simulink model "W01_Base_MapUnrealPb_cs"  (R2019a)
settings: Solver=FixedStepDiscrete  StartTime=0.0  StopTime=100  FixedStep=1/20  RelTol=1e-3
PreLoadFcn:
  | mbxruntime.callbacks.PreLoadFcn(bdroot);
  | check_NUTS_defined
  | model_closed = 0;
  | assignin('base',['model_closed_' bdroot],false);
PostLoadFcn:
  | mbxruntime.callbacks.PostLoadFcn(bdroot);
InitFcn:
  | mbxruntime.callbacks.InitFcn(bdroot);
StartFcn:
  | mbxruntime.callbacks.StartFcn(bdroot);
StopFcn:
  | mbxruntime.callbacks.StopFcn(bdroot);;
  | 
model workspace: external: MAT-File .\W01_Base_MapUnrealPb_cs_hws.mat (data not in the file)
undefined symbols (not defined in the file or in its folder): DiscIntNeverNeededParam, Header, InitImageOutputDir, mbxruntime, Orientation, Poses, Poses_SL_Info, Position, tabledata, W01_Base_MapUnrealPb_cs_1fa864f6888febdf, W01_Base_MapUnrealPb_cs_363eba12a3b1b1b2, W01_Base_MapUnrealPb_cs_37eda8bac69b475f, W01_Base_MapUnrealPb_cs_40adcda03182ca89, W01_Base_MapUnrealPb_cs_44a3a79c674e7cb2, W01_Base_MapUnrealPb_cs_46a8a6a698ab1958, W01_Base_MapUnrealPb_cs_4b9c3713e3f2fd86, W01_Base_MapUnrealPb_cs_5c6746169321700b, W01_Base_MapUnrealPb_cs_86551b8b23c33892, W01_Base_MapUnrealPb_cs_8a63c705da999788, W01_Base_MapUnrealPb_cs_Audi_A8_Sedan_1_Path_pathUniqueID, W01_Base_MapUnrealPb_cs_c83488546359e010, W01_Base_MapUnrealPb_cs_Child_RegularAni_1_Path_pathUniqueID, W01_Base_MapUnrealPb_cs_Child_RegularAni_2_Path_pathUniqueID, W01_Base_MapUnrealPb_cs_e51f5c648b171aa6, W01_Base_MapUnrealPb_cs_e7dea57c46773520, W01_Base_MapUnrealPb_cs_ea4bc0bfbb614fa1, W01_Base_MapUnrealPb_cs_Female_RegularAni_1_Path_pathUniqueID, W01_Base_MapUnrealPb_cs_Male_RegularAni_1_Path_pathUniqueID, W01_Base_MapUnrealPb_cs_Male_RegularAni_2_Path_pathUniqueID
libraries: adeye_lib x46, simulink_extras x30, simulink x10, robotlib x4, sharedtransform x2, PreScanSimulinkLibrary x2, PreScanUsefulBlocks x1
(part 1 of 9)
CloseFcn:
  | mbxruntime.callbacks.CloseFcn(bdroot);
  | evalin('base',['clear model_closed_' bdroot]);
  | model_closed = 1;
settings Model: Creator=PRESCAN  LastModifiedBy=adeye
settings DataIOCC: LimitDataPoints=on  SaveFormat=Array  SignalLoggingSaveFormat=ModelDataLogs  ReturnWorkspaceOutputs=off
settings OptimizationCC: DefaultParameterBehavior=Inlined  ExpressionDepthLimit=2147483647  InitFltsAndDblsToZero=on  LifeSpan=inf
settings DebuggingCC: SaveWithParameterizedLinksMsg=none  UnderspecifiedInitializationDetection=Classic  MergeDetectMultiDrivingBlocksExec=none  SignalResolutionControl=TryResolveAllWithWarning  MultiTaskDSMMsg=warning  MultiTaskCondExecSysMsg=none  FcnCallInpInsideContextMsg=warning  StateNameClashWarn=warning  SFUnexpectedBacktrackingDiag=warning  SFNoUnconditionalDefaultTransitionDiag=warning  SFExecutionAtInitializationDiag=none  ArithmeticOperatorsInVariantConditions=warning
settings HardwareCC: ProdBitPerPointer=32  ProdBitPerSizeT=32  ProdBitPerPtrDiffT=32  ProdLargestAtomicFloat=None  ProdIntDivRoundTo=Undefined  ProdEndianess=Unspecified  ProdWordSize=32  ProdHWDeviceType=32-bit Generic
settings ModelReferenceCC: UpdateModelReferenceTargets=IfOutOfDate  PropagateSignalLabelsOutOfModel=off
settings SFSimCC: SimUseLocalCustomCode=off  SimParseCustomCode=off
settings SFSimCC: SimCustomHeaderCode=|
  | #include "prescan.h"
  | #include "prescan_platform.h"
  | #include "prescan_aimsunturnindicatorsetter_data.h"
settings RTWCC: RTWUseLocalCustomCode=off
settings CodeAppCC: StateflowObjectComments=on
settings GRTTargetCC: TargetFcnLib=ansi_tfl_tmw.mat  TargetLangStandard=C89/C90 (ANSI)  GeneratePreprocessorConditionals=Disable all  CombineOutputUpdateFcns=off  GRTInterface=on
settings ConfigComp: CovMetricSettings=dw  CovHtmlReporting=on  CovSaveCumulativeToWorkspaceVar=on  CovSaveSingleToWorkspaceVar=on  CovExternalEMLEnable=off  CovSFcnEnable=off

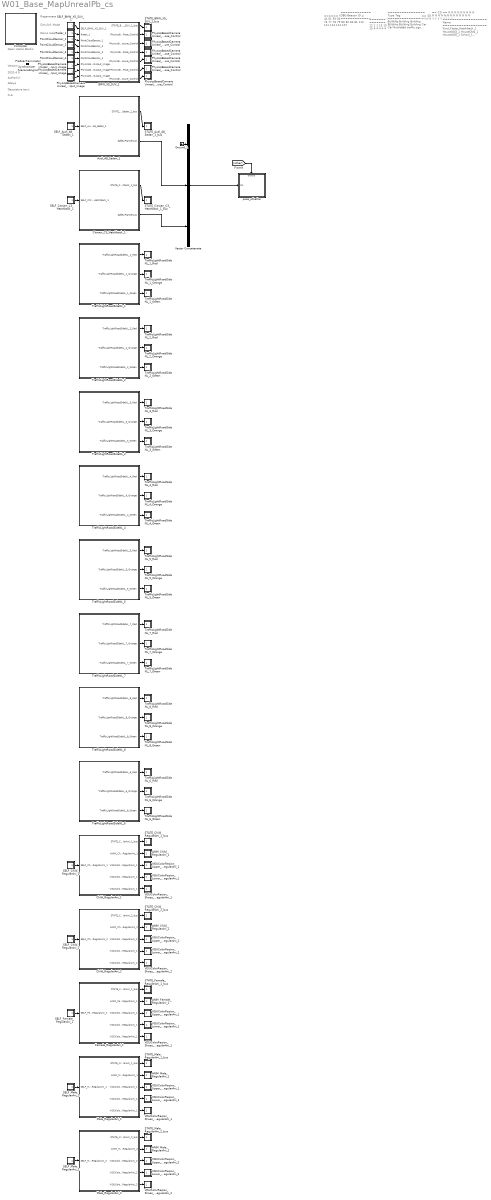
== system W01_Base_MapUnrealPb_cs ==
  note: Regenerate
  note: Simulink Mode
  note: Open Useful Blocks
  note: 2020.4.0
  note: Version:
  note: Author(s):
  note: Adeye
  note: Descriptive text:
  note: N.A.
  note: Demo Help
  note: ======
      | Num ID
      | ======
      | 44
      | 91
      | 93
      | 94
      | 95
      | 96
      | 97
      | 102
      | 108
      | 76
      | 77
      | 78
      | 79
      | 80
      | 82
      | 83
      | 81
      | 112
      | 111
      | 113
      | 114
      | 107
  note: =============
      | OBU-Beacon ID
      | =============
  note: =======
      | Type ID
      | =======
      | 1
      | 12
      | 12
      | 12
      | 12
      | 12
      | 12
      | 1
      | 1
      | 15
      | 15
      | 15
      | 15
      | 15
      | 15
      | 15
      | 15
      | 4
      | 4
      | 4
      | 4
      | 4
  note: ================
      | Type Tag
      | ================
      | Car
      | Building
      | Building
      | Building
      | Building
      | Building
      | Building
      | Car
      | Car
      | Animated traffic sign
      | Animated traffic sign
      | Animated traffic sign
      | Animated traffic sign
      | Animated traffic sign
      | Animated traffic sign
      | Animated traffic sign
      | Animated traffic sign
      | Human
      | Human
      | Human
      | Human
      | Human
  note: ==
      | SD
      | ==
      | Y
      | Y
      | Y
      | Y
      | Y
      | Y
      | Y
      | Y
      | Y
      | Y
      | Y
      | Y
      | Y
      | Y
      | Y
      | Y
      | Y
      | Y
      | Y
      | Y
      | Y
      | Y
  note: ==
      | CD
      | ==
      | N
      | N
      | N
      | N
      | N
      | N
      | N
      | N
      | N
      | N
      | N
      | N
      | N
      | N
      | N
      | N
      | N
      | N
      | N
      | N
      | N
      | N
  note: ===================
      | Name
      | ===================
      | Ford_Fiesta_Hatchback_1
      | HouseOld3_1
      | HouseOld4_1
      | HouseOld5_1
      | School_1
      | OfficeBrownFlat_1
      | OfficeBrownTall2_1
      | Audi_A8_Sedan_1
      | Citroen_C3_Hatchback_1
      | TrafficLightRoadSideNL_1
      | TrafficLightRoadSideNL_2
      | TrafficLightRoadSideNL_3
      | TrafficLightRoadSideNL_4
      | TrafficLightRoadSideNL_5
      | TrafficLightRoadSideNL_7
      | TrafficLightRoadSideNL_8
      | TrafficLightRoadSideNL_6
      | Child_RegularAni_1
      | Child_RegularAni_2
      | Female_RegularAni_1
      | Male_RegularAni_1
      | Male_RegularAni_2
  ANIM_Child_RegularAni_1 : Subsystem  Tag=actuator/AnimationOutport  Priority=0  LoadFcn=load('PreScanAnimActuatorData.mat')  mask(PreScan Sink Block: State Animation){}
      mask help: The Human Animation port allows the human to walk, run or bend
      settings: OpenFcn=open_system([gcb '/Actuator'],'mask')
      mask Help: eval('openHelp(239)')
      mask Display: image(imread('HumanAnimated.jpg'))
  ANIM_Child_RegularAni_2 : Subsystem  Tag=actuator/AnimationOutport  Priority=0  LoadFcn=load('PreScanAnimActuatorData.mat')  mask(PreScan Sink Block: State Animation){}
      mask help: The Human Animation port allows the human to walk, run or bend
      settings: OpenFcn=open_system([gcb '/Actuator'],'mask')
      mask Help: eval('openHelp(239)')
      mask Display: image(imread('HumanAnimated.jpg'))
  ANIM_Female_RegularAni_1 : Subsystem  Tag=actuator/AnimationOutport  Priority=0  LoadFcn=load('PreScanAnimActuatorData.mat')  mask(PreScan Sink Block: State Animation){}
      mask help: The Human Animation port allows the human to walk, run or bend
      settings: OpenFcn=open_system([gcb '/Actuator'],'mask')
      mask Help: eval('openHelp(239)')
      mask Display: image(imread('HumanAnimated.jpg'))
  ANIM_Male_RegularAni_1 : Subsystem  Tag=actuator/AnimationOutport  Priority=0  LoadFcn=load('PreScanAnimActuatorData.mat')  mask(PreScan Sink Block: State Animation){}
      mask help: The Human Animation port allows the human to walk, run or bend
      settings: OpenFcn=open_system([gcb '/Actuator'],'mask')
      mask Help: eval('openHelp(239)')
      mask Display: image(imread('HumanAnimated.jpg'))
  ANIM_Male_RegularAni_2 : Subsystem  Tag=actuator/AnimationOutport  Priority=0  LoadFcn=load('PreScanAnimActuatorData.mat')  mask(PreScan Sink Block: State Animation){}
      mask help: The Human Animation port allows the human to walk, run or bend
      settings: OpenFcn=open_system([gcb '/Actuator'],'mask')
      mask Help: eval('openHelp(239)')
      mask Display: image(imread('HumanAnimated.jpg'))
  Audi_A8_Sedan_1 : Subsystem  Tag=WorldObjectSubSystem  InitFcn=UniqueId = '18645';
      mask init:
      | modelPath = GenericModelHelper.getGenericModelFilePath('ModelDepo','Vehicles\Audi_A8\Audi_A8.pgmb','e33fe1ddcf3e8ae97caccbc8f2fa74ac');imagePath = GenericModelHelper.getCompilationPicture(modelPath, 'Audi_A8_HighPoly.png');
      mask Display: image(imread(imagePath));color('white');text(0, 0, ' ID=102\n')
  BMW_X5_SUV_1 : Subsystem  Tag=WorldObjectSubSystem  InitFcn=UniqueId = '9040';
      mask init:
      | modelPath = GenericModelHelper.getGenericModelFilePath('ModelDepo','Vehicles\BMW_X5\BMW_X5.pgmb','bfeb1c11467705ab888b3011684c848b');imagePath = GenericModelHelper.getCompilationPicture(modelPath, 'BMW_X5_HighPoly.png');
      mask Display: image(imread(imagePath));color('white');text(0, 0, ' ID=55\n')
  Child_RegularAni_1 : Subsystem  Tag=WorldObjectSubSystem  InitFcn=UniqueId = '18395';
      mask init:
      | modelPath = GenericModelHelper.getGenericModelFilePath('ModelDepo','Humans\ChildRegular\Child_Regular.pgmb','0405fb6e1c51d7af34e60031bef9e83f');imagePath = GenericModelHelper.getCompilationPicture(modelPath, 'ChildRegular.png');
      mask Display: image(imread(imagePath));color('white');text(0, 0, ' ID=112\n')
  Child_RegularAni_2 : Subsystem  Tag=WorldObjectSubSystem  InitFcn=UniqueId = '18628';
      mask init: same as W01_Base_MapUnrealPb_cs/Child_RegularAni_1
      mask Display: image(imread(imagePath));color('white');text(0, 0, ' ID=111\n')
  Citroen_C3_Hatchback_1 : Subsystem  Tag=WorldObjectSubSystem  InitFcn=UniqueId = '18857';
      mask init:
      | modelPath = GenericModelHelper.getGenericModelFilePath('ModelDepo','Vehicles\Citroen_C3\Citroen_C3.pgmb','e804ced06d50dbfc6a2202ab3ad01b0c');imagePath = GenericModelHelper.getCompilationPicture(modelPath, 'Citroen_C3_HighPoly.png');
      mask Display: image(imread(imagePath));color('white');text(0, 0, ' ID=108\n')
  Controller : Subsystem  Description=8A3CD2955739A82C886C20AE3E253D78460D53180EE2C1B14CC08DF75A70BE77  Priority=-1  LoadFcn=load PreScanControllerData  mask(PreScan Simulation Controller){prescanversion='2020.4.0', ModelReferencing=off, TimeStep=1/20, ControlMode=0, PreScanExecutionMode=on, ControllerCount=0, ControllerIndex=0, ControllerOptions=''}
      mask prompts: prescanversion "PreScan Version"; ModelReferencing "Use Model Referencing"; TimeStep "Upload Period [s]"; ControlMode "Control Mode"; PreScanExecutionMode "Execution Mode"; ControllerCount "Controller Count"; ControllerIndex "Controller Index"; ControllerOptions "Controller Options"
      mask help:
      | Please do not remove this block from the compilation sheet,
      | as it connects the model to the PreScan environment.
      mask init:
      | model = bdroot(gcb);
      | ExperimentFile = mbxruntime.findExperimentFile(model,true); %relative path
      | 
      | [d1, d2, d3, prescandata] = prescan_Settings();
      | ModelDepo = fullfile(prescandata,'ModelDepo'); 
      | 
      | RTmode = mbxruntime.getRTMode(model);
      | 
      | SimulationMode = get_param(bdroot,'SimulationMode');
      | if strcmp(SimulationMode, 'rapid-accelerator')
      |     SimulationMode = 'external';
      | end
      | TargetName = get_param(bdroot,'SystemTargetFile');
      settings: ModelCloseFcn=assignin('base',['model_closed_' bdroot],true);
      mask Help: eval('openHelp(812)')
      mask Display: image(imread('prescanlogo.ico'))
  Female_RegularAni_1 : Subsystem  Tag=WorldObjectSubSystem  InitFcn=UniqueId = '18631';
      mask init:
      | modelPath = GenericModelHelper.getGenericModelFilePath('ModelDepo','Humans\FemaleRegular\Female_Regular.pgmb','a60942a07dc01011c3a5e5a36c910370');imagePath = GenericModelHelper.getCompilationPicture(modelPath, 'FemaleRegular.png');
      mask Display: image(imread(imagePath));color('white');text(0, 0, ' ID=113\n')
  Ground_1 : Ground
  Male_RegularAni_1 : Subsystem  Tag=WorldObjectSubSystem  InitFcn=UniqueId = '18634';
      mask init:
      | modelPath = GenericModelHelper.getGenericModelFilePath('ModelDepo','Humans\MaleRegular\Male_Regular.pgmb','f91824e3173f6a1007ae98b99b2fb1bd');imagePath = GenericModelHelper.getCompilationPicture(modelPath, 'MaleRegular.png');
      mask Display: image(imread(imagePath));color('white');text(0, 0, ' ID=114\n')
  Male_RegularAni_2 : Subsystem  Tag=WorldObjectSubSystem  InitFcn=UniqueId = '18853';
      mask init: same as W01_Base_MapUnrealPb_cs/Male_RegularAni_1
      mask Display: image(imread(imagePath));color('white');text(0, 0, ' ID=107\n')
  PhysicsBasedCameraUnreal_1_ImageRGBOutput_image : Subsystem  Tag=sensor/plugin/sfun_PBCURGBOutput  Priority=30  mask(PreScan Source Block: Camera Sensor){}
      mask help: Unreal Camera ImageRGBOutput image
      settings: OpenFcn=open_system([gcb '/Sensor'],'mask')
      mask Help: eval('openHelp()')
      mask Display: image(imread('CameraSensor.png'))
  PhysicsBasedCameraUnreal_1_PBCUExposure_Control : Subsystem  Tag=actuator/plugin/sfun_PBCUExposure  Priority=0  mask(Physics Based Camera (Unreal) plugin block){}
      mask help: PBCU Control I/O
      settings: OpenFcn=open_system([gcb '/Actuator'],'mask')
      mask Help: eval('openHelp()')
      mask Display: image(imread('ico_PBCUControl.png'))
  PhysicsBasedCameraUnreal_1_PBCUPose_Control : Subsystem  Tag=actuator/plugin/sfun_PBCUPose  Priority=0  mask(Physics Based Camera (Unreal) plugin block){}
      mask help: PBCU Control I/O
      settings: OpenFcn=open_system([gcb '/Actuator'],'mask')
      mask Help: eval('openHelp()')
      mask Display: image(imread('ico_PBCUControl.png'))
  PhysicsBasedCameraUnreal_2_ImageRGBOutput_image : Subsystem  Tag=sensor/plugin/sfun_PBCURGBOutput  Priority=30  mask(PreScan Source Block: Camera Sensor){}
      mask help: Unreal Camera ImageRGBOutput image
      settings: OpenFcn=open_system([gcb '/Sensor'],'mask')
      mask Help: eval('openHelp()')
      mask Display: image(imread('CameraSensor.png'))
  PhysicsBasedCameraUnreal_2_PBCUExposure_Control : Subsystem  Tag=actuator/plugin/sfun_PBCUExposure  Priority=0  mask(Physics Based Camera (Unreal) plugin block){}
      mask help: PBCU Control I/O
      settings: OpenFcn=open_system([gcb '/Actuator'],'mask')
      mask Help: eval('openHelp()')
      mask Display: image(imread('ico_PBCUControl.png'))
  PhysicsBasedCameraUnreal_2_PBCUPose_Control : Subsystem  Tag=actuator/plugin/sfun_PBCUPose  Priority=0  mask(Physics Based Camera (Unreal) plugin block){}
      mask help: PBCU Control I/O
      settings: OpenFcn=open_system([gcb '/Actuator'],'mask')
      mask Help: eval('openHelp()')
      mask Display: image(imread('ico_PBCUControl.png'))
  PhysicsBasedCameraUnreal_3_ImageRGBOutput_image : Subsystem  Tag=sensor/plugin/sfun_PBCURGBOutput  Priority=30  mask(PreScan Source Block: Camera Sensor){}
      mask help: Unreal Camera ImageRGBOutput image
      settings: OpenFcn=open_system([gcb '/Sensor'],'mask')
      mask Help: eval('openHelp()')
      mask Display: image(imread('CameraSensor.png'))
  PhysicsBasedCameraUnreal_3_PBCUExposure_Control : Subsystem  Tag=actuator/plugin/sfun_PBCUExposure  Priority=0  mask(Physics Based Camera (Unreal) plugin block){}
      mask help: PBCU Control I/O
      settings: OpenFcn=open_system([gcb '/Actuator'],'mask')
      mask Help: eval('openHelp()')
      mask Display: image(imread('ico_PBCUControl.png'))
  PhysicsBasedCameraUnreal_3_PBCUPose_Control : Subsystem  Tag=actuator/plugin/sfun_PBCUPose  Priority=0  mask(Physics Based Camera (Unreal) plugin block){}
      mask help: PBCU Control I/O
      settings: OpenFcn=open_system([gcb '/Actuator'],'mask')
      mask Help: eval('openHelp()')
      mask Display: image(imread('ico_PBCUControl.png'))
  PointCloudSensor_1 : Subsystem  Tag=sensor/PointCloudInport  Priority=30  mask(PreScan Source Block: Point Cloud Sensor){}
      mask help: The Point Cloud Sensor provides XYZ positions relative to the sensor
      settings: OpenFcn=open_system([gcb '/Sensor'],'mask')
      mask Help: eval('openHelp(6400)')
      mask Display: image(imread('PointCloudSensorSL.png'))
  PointCloudSensor_2 : Subsystem  Tag=sensor/PointCloudInport  Priority=30  mask(PreScan Source Block: Point Cloud Sensor){}
      mask help: The Point Cloud Sensor provides XYZ positions relative to the sensor
      settings: OpenFcn=open_system([gcb '/Sensor'],'mask')
      mask Help: eval('openHelp(6400)')
      mask Display: image(imread('PointCloudSensorSL.png'))
  PointCloudSensor_3 : Subsystem  Tag=sensor/PointCloudInport  Priority=30  mask(PreScan Source Block: Point Cloud Sensor){}
      mask help: The Point Cloud Sensor provides XYZ positions relative to the sensor
      settings: OpenFcn=open_system([gcb '/Sensor'],'mask')
      mask Help: eval('openHelp(6400)')
      mask Display: image(imread('PointCloudSensorSL.png'))
  PointCloudSensor_4 : Subsystem  Tag=sensor/PointCloudInport  Priority=30  mask(PreScan Source Block: Point Cloud Sensor){}
      mask help: The Point Cloud Sensor provides XYZ positions relative to the sensor
      settings: OpenFcn=open_system([gcb '/Sensor'],'mask')
      mask Help: eval('openHelp(6400)')
      mask Display: image(imread('PointCloudSensorSL.png'))
  PreScanTerminator : Subsystem  Tag=PreScanTerminator  Priority=999  LoadFcn=load PrescanTerminatorData  mask(PreScan Simulation Terminator){TimeStep=1/20}
      mask prompts: TimeStep "Upload Period [s]"
      mask help:
      | Please do not remove this block from the compilation sheet as it
      | connects the model to the PreScan environment.
      mask Help: eval('openHelp(812)')
      mask Display: image(imread('prescanlogo.ico'))
  Radar_1 : Subsystem  Tag=sensor/Radar  Priority=30  LoadFcn=load('PrescanScannerSensorData.mat');load('PrescanScannerSensorMessage.mat')  mask(PreScan Source Block: Radar Sensor){}
      mask help:
      | The Radar Sensor is a detailed sensor based on a physical radar
      | model that includes Antenna GAIN Maps (AGM) and atmospheric
      | attenuation.
      |
      | For more information, please click Help.
      settings: OpenFcn=open_system([gcb '/Sensor'],'mask')
      mask Help: eval('openHelp(1464)')
      mask Display: image(imread('Radar.png'))
  SELF_Audi_A8_Sedan_1 : Subsystem  Tag=sensor/SelfPort  Priority=30  LoadFcn=load('PreScanSelfSensorData.mat')  mask(PreScan Source Block: SELF){}
      mask help:
      | The SELF port shows (state) information of the actor itself. The outputs are position in the experiment's axis system and the GPS coordinates, and the object's absolute velocity and compass heading.
      |
      | For more information, please click Help.
      settings: OpenFcn=open_system([gcb '/Sensor'],'mask')
      mask Help: eval('openHelp(462)')
      mask Display: image(imread('GPS.png'))
  SELF_BMW_X5_SUV_1 : Subsystem  Tag=sensor/SelfPort  Priority=30  LoadFcn=load('PreScanSelfSensorData.mat')  mask(PreScan Source Block: SELF){}
      mask help:
      | The SELF port shows (state) information of the actor itself. The outputs are position in the experiment's axis system and the GPS coordinates, and the object's absolute velocity and compass heading.
      |
      | For more information, please click Help.
      settings: OpenFcn=open_system([gcb '/Sensor'],'mask')
      mask Help: eval('openHelp(462)')
      mask Display: image(imread('GPS.png'))
  SELF_Child_RegularAni_1 : Subsystem  Tag=sensor/SelfPort  Priority=30  LoadFcn=load('PreScanSelfSensorData.mat')  mask(PreScan Source Block: SELF){}
      mask help:
      | The SELF port shows (state) information of the actor itself. The outputs are position in the experiment's axis system and the GPS coordinates, and the object's absolute velocity and compass heading.
      |
      | For more information, please click Help.
      settings: OpenFcn=open_system([gcb '/Sensor'],'mask')
      mask Help: eval('openHelp(462)')
      mask Display: image(imread('GPS.png'))
  SELF_Child_RegularAni_2 : Subsystem  Tag=sensor/SelfPort  Priority=30  LoadFcn=load('PreScanSelfSensorData.mat')  mask(PreScan Source Block: SELF){}
      mask help:
      | The SELF port shows (state) information of the actor itself. The outputs are position in the experiment's axis system and the GPS coordinates, and the object's absolute velocity and compass heading.
      |
      | For more information, please click Help.
      settings: OpenFcn=open_system([gcb '/Sensor'],'mask')
      mask Help: eval('openHelp(462)')
      mask Display: image(imread('GPS.png'))
  SELF_Citroen_C3_Hatchback_1 : Subsystem  Tag=sensor/SelfPort  Priority=30  LoadFcn=load('PreScanSelfSensorData.mat')  mask(PreScan Source Block: SELF){}
      mask help:
      | The SELF port shows (state) information of the actor itself. The outputs are position in the experiment's axis system and the GPS coordinates, and the object's absolute velocity and compass heading.
      |
      | For more information, please click Help.
      settings: OpenFcn=open_system([gcb '/Sensor'],'mask')
      mask Help: eval('openHelp(462)')
      mask Display: image(imread('GPS.png'))
  SELF_Female_RegularAni_1 : Subsystem  Tag=sensor/SelfPort  Priority=30  LoadFcn=load('PreScanSelfSensorData.mat')  mask(PreScan Source Block: SELF){}
      mask help:
      | The SELF port shows (state) information of the actor itself. The outputs are position in the experiment's axis system and the GPS coordinates, and the object's absolute velocity and compass heading.
      |
      | For more information, please click Help.
      settings: OpenFcn=open_system([gcb '/Sensor'],'mask')
      mask Help: eval('openHelp(462)')
      mask Display: image(imread('GPS.png'))
  SELF_Male_RegularAni_1 : Subsystem  Tag=sensor/SelfPort  Priority=30  LoadFcn=load('PreScanSelfSensorData.mat')  mask(PreScan Source Block: SELF){}
      mask help:
      | The SELF port shows (state) information of the actor itself. The outputs are position in the experiment's axis system and the GPS coordinates, and the object's absolute velocity and compass heading.
      |
      | For more information, please click Help.
      settings: OpenFcn=open_system([gcb '/Sensor'],'mask')
      mask Help: eval('openHelp(462)')
      mask Display: image(imread('GPS.png'))
  SELF_Male_RegularAni_2 : Subsystem  Tag=sensor/SelfPort  Priority=30  LoadFcn=load('PreScanSelfSensorData.mat')  mask(PreScan Source Block: SELF){}
      mask help:
      | The SELF port shows (state) information of the actor itself. The outputs are position in the experiment's axis system and the GPS coordinates, and the object's absolute velocity and compass heading.
      |
      | For more information, please click Help.
      settings: OpenFcn=open_system([gcb '/Sensor'],'mask')
      mask Help: eval('openHelp(462)')
      mask Display: image(imread('GPS.png'))
  STATE_Audi_A8_Sedan_1_bus : Subsystem  Tag=actuator/StatePort  Priority=0  LoadFcn=load('PreScanStateActuatorData.mat')  mask(PreScan Sink Block: State){}
      mask help:
      | The Actor State contains a vector signal of size (9x1), containing the following signals:
      |
      | -  Position    	(x,y,z)             	[m]
      | -  Velocity    	(vx,vy,vz)         	[m/s]
      | -  Angles       	(Roll, Pitch, Yaw)	[rad]
      |
      | The Actor state is defined in the global axis system.
      | The state is superponed on the Initial position defined in the GUI.
      |
      | For more information, please click Help.
      settings: OpenFcn=open_system([gcb '/Actuator'],'mask')
      mask Help: eval('openHelp(222)')
      mask Display: image(imread('State.png'))
  STATE_BMW_X5_SUV_1_bus : Subsystem  Tag=actuator/StatePort  Priority=0  LoadFcn=load('PreScanStateActuatorData.mat')  mask(PreScan Sink Block: State){}
      mask help:
      | The Actor State contains a vector signal of size (9x1), containing the following signals:
      |
      | -  Position    	(x,y,z)             	[m]
      | -  Velocity    	(vx,vy,vz)         	[m/s]
      | -  Angles       	(Roll, Pitch, Yaw)	[rad]
      |
      | The Actor state is defined in the global axis system.
      | The state is superponed on the Initial position defined in the GUI.
      |
      | For more information, please click Help.
      settings: OpenFcn=open_system([gcb '/Actuator'],'mask')
      mask Help: eval('openHelp(222)')
      mask Display: image(imread('State.png'))
  STATE_Child_RegularAni_1_bus : Subsystem  Tag=actuator/StatePort  Priority=0  LoadFcn=load('PreScanStateActuatorData.mat')  mask(PreScan Sink Block: State){}
      mask help:
      | The Actor State contains a vector signal of size (9x1), containing the following signals:
      |
      | -  Position    	(x,y,z)             	[m]
      | -  Velocity    	(vx,vy,vz)         	[m/s]
      | -  Angles       	(Roll, Pitch, Yaw)	[rad]
      |
      | The Actor state is defined in the global axis system.
      | The state is superponed on the Initial position defined in the GUI.
      |
      | For more information, please click Help.
      settings: OpenFcn=open_system([gcb '/Actuator'],'mask')
      mask Help: eval('openHelp(222)')
      mask Display: image(imread('State.png'))
  STATE_Child_RegularAni_2_bus : Subsystem  Tag=actuator/StatePort  Priority=0  LoadFcn=load('PreScanStateActuatorData.mat')  mask(PreScan Sink Block: State){}
      mask help:
      | The Actor State contains a vector signal of size (9x1), containing the following signals:
      |
      | -  Position    	(x,y,z)             	[m]
      | -  Velocity    	(vx,vy,vz)         	[m/s]
      | -  Angles       	(Roll, Pitch, Yaw)	[rad]
      |
      | The Actor state is defined in the global axis system.
      | The state is superponed on the Initial position defined in the GUI.
      |
      | For more information, please click Help.
      settings: OpenFcn=open_system([gcb '/Actuator'],'mask')
      mask Help: eval('openHelp(222)')
      mask Display: image(imread('State.png'))
  STATE_Citroen_C3_Hatchback_1_bus : Subsystem  Tag=actuator/StatePort  Priority=0  LoadFcn=load('PreScanStateActuatorData.mat')  mask(PreScan Sink Block: State){}
      mask help:
      | The Actor State contains a vector signal of size (9x1), containing the following signals:
      |
      | -  Position    	(x,y,z)             	[m]
      | -  Velocity    	(vx,vy,vz)         	[m/s]
      | -  Angles       	(Roll, Pitch, Yaw)	[rad]
      |
      | The Actor state is defined in the global axis system.
      | The state is superponed on the Initial position defined in the GUI.
      |
      | For more information, please click Help.
      settings: OpenFcn=open_system([gcb '/Actuator'],'mask')
      mask Help: eval('openHelp(222)')
      mask Display: image(imread('State.png'))
  STATE_Female_RegularAni_1_bus : Subsystem  Tag=actuator/StatePort  Priority=0  LoadFcn=load('PreScanStateActuatorData.mat')  mask(PreScan Sink Block: State){}
      mask help:
      | The Actor State contains a vector signal of size (9x1), containing the following signals:
      |
      | -  Position    	(x,y,z)             	[m]
      | -  Velocity    	(vx,vy,vz)         	[m/s]
      | -  Angles       	(Roll, Pitch, Yaw)	[rad]
      |
      | The Actor state is defined in the global axis system.
      | The state is superponed on the Initial position defined in the GUI.
      |
      | For more information, please click Help.
      settings: OpenFcn=open_system([gcb '/Actuator'],'mask')
      mask Help: eval('openHelp(222)')
      mask Display: image(imread('State.png'))
  STATE_Male_RegularAni_1_bus : Subsystem  Tag=actuator/StatePort  Priority=0  LoadFcn=load('PreScanStateActuatorData.mat')  mask(PreScan Sink Block: State){}
      mask help:
      | The Actor State contains a vector signal of size (9x1), containing the following signals:
      |
      | -  Position    	(x,y,z)             	[m]
      | -  Velocity    	(vx,vy,vz)         	[m/s]
      | -  Angles       	(Roll, Pitch, Yaw)	[rad]
      |
      | The Actor state is defined in the global axis system.
      | The state is superponed on the Initial position defined in the GUI.
      |
      | For more information, please click Help.
      settings: OpenFcn=open_system([gcb '/Actuator'],'mask')
      mask Help: eval('openHelp(222)')
      mask Display: image(imread('State.png'))
  STATE_Male_RegularAni_2_bus : Subsystem  Tag=actuator/StatePort  Priority=0  LoadFcn=load('PreScanStateActuatorData.mat')  mask(PreScan Sink Block: State){}
      mask help:
      | The Actor State contains a vector signal of size (9x1), containing the following signals:
      |
      | -  Position    	(x,y,z)             	[m]
      | -  Velocity    	(vx,vy,vz)         	[m/s]
      | -  Angles       	(Roll, Pitch, Yaw)	[rad]
      |
      | The Actor state is defined in the global axis system.
      | The state is superponed on the Initial position defined in the GUI.
      |
      | For more information, please click Help.
      settings: OpenFcn=open_system([gcb '/Actuator'],'mask')
      mask Help: eval('openHelp(222)')
      mask Display: image(imread('State.png'))
  ScenarioEngine : Subsystem  Tag=PreScanOpenScenarioBlock  Priority=10  LoadFcn=load PrescanSynchronizeData  mask(PreScan Simulation Core Block){TimeStep=1/20}
      mask prompts: TimeStep "Timestep [s]"
      mask help:
      | Please do not remove this block from the PreScan compilation sheet,
      | as it contains essential configuration parameters for a PreScan simulation.
      settings: DeleteFcn=PreScanBlockDeleteFcn;
      mask Display: image(imread('prescanlogo.ico'))
  Synchronizer : Subsystem  Tag=PreScanSynchronizer  Priority=20  LoadFcn=load PrescanSynchronizeData  mask(PreScan Simulation Core Block){TimeStep=1/20}
      mask prompts: TimeStep "Timestep [s]"
      mask help:
      | Please do not remove this block from the PreScan compilation sheet,
      | as it contains essential configuration parameters for a PreScan simulation.
      settings: DeleteFcn=PreScanBlockDeleteFcn;
      mask Display: image(imread('prescanlogo.ico'))
  TrafficLightRoadSideNL_1 : Subsystem  Tag=WorldObjectSubSystem  InitFcn=UniqueId = '646';
      mask init:
      | modelPath = GenericModelHelper.getGenericModelFilePath('ModelDepo','AnimatedElements\TrafficLight_NL\Roadside\Roadside_NL.pgmb','2000fba5e1a6d0fba32e88146243c3cb');imagePath = GenericModelHelper.getCompilationPicture(modelPath, 'Roadside_NL.png');
      mask Display: image(imread(imagePath));color('white');text(0, 0, ' ID=76\n')
  TrafficLightRoadSideNL_1_Green : Subsystem  Tag=actuator/Green  Priority=0  LoadFcn=load('PreScanVisuLightActuatorData');load('PrescanRPYData');load('PrescanXYZData');load('PreScanRGBData')  mask(PreScan Sink Block: VisuActiveLight){}
      mask help:
      | The VisuActiveLight block provides a way for detailed animation of Light Sources, such as the indicator, brake, fog and main lights of a vehicle, or a light post.
      |
      | For more information, please click Help.
      settings: OpenFcn=open_system([gcb '/Actuator'],'mask')
      mask Help: eval('openHelp(209)')
      mask Display: image(imread('HeadLight.png'))
  TrafficLightRoadSideNL_1_Orange : Subsystem  Tag=actuator/Orange  Priority=0  LoadFcn=load('PreScanVisuLightActuatorData');load('PrescanRPYData');load('PrescanXYZData');load('PreScanRGBData')  mask(PreScan Sink Block: VisuActiveLight){}
      mask help:
      | The VisuActiveLight block provides a way for detailed animation of Light Sources, such as the indicator, brake, fog and main lights of a vehicle, or a light post.
      |
      | For more information, please click Help.
      settings: OpenFcn=open_system([gcb '/Actuator'],'mask')
      mask Help: eval('openHelp(209)')
      mask Display: image(imread('HeadLight.png'))
  TrafficLightRoadSideNL_1_Red : Subsystem  Tag=actuator/Red  Priority=0  LoadFcn=load('PreScanVisuLightActuatorData');load('PrescanRPYData');load('PrescanXYZData');load('PreScanRGBData')  mask(PreScan Sink Block: VisuActiveLight){}
      mask help:
      | The VisuActiveLight block provides a way for detailed animation of Light Sources, such as the indicator, brake, fog and main lights of a vehicle, or a light post.
      |
      | For more information, please click Help.
      settings: OpenFcn=open_system([gcb '/Actuator'],'mask')
      mask Help: eval('openHelp(209)')
      mask Display: image(imread('HeadLight.png'))
  TrafficLightRoadSideNL_2 : Subsystem  Tag=WorldObjectSubSystem  InitFcn=UniqueId = '647';
      mask init: same as W01_Base_MapUnrealPb_cs/TrafficLightRoadSideNL_1
      mask Display: image(imread(imagePath));color('white');text(0, 0, ' ID=77\n')
  TrafficLightRoadSideNL_2_Green : Subsystem  Tag=actuator/Green  Priority=0  LoadFcn=load('PreScanVisuLightActuatorData');load('PrescanRPYData');load('PrescanXYZData');load('PreScanRGBData')  mask(PreScan Sink Block: VisuActiveLight){}
      mask help:
      | The VisuActiveLight block provides a way for detailed animation of Light Sources, such as the indicator, brake, fog and main lights of a vehicle, or a light post.
      |
      | For more information, please click Help.
      settings: OpenFcn=open_system([gcb '/Actuator'],'mask')
      mask Help: eval('openHelp(209)')
      mask Display: image(imread('HeadLight.png'))
  TrafficLightRoadSideNL_2_Orange : Subsystem  Tag=actuator/Orange  Priority=0  LoadFcn=load('PreScanVisuLightActuatorData');load('PrescanRPYData');load('PrescanXYZData');load('PreScanRGBData')  mask(PreScan Sink Block: VisuActiveLight){}
      mask help:
      | The VisuActiveLight block provides a way for detailed animation of Light Sources, such as the indicator, brake, fog and main lights of a vehicle, or a light post.
      |
      | For more information, please click Help.
      settings: OpenFcn=open_system([gcb '/Actuator'],'mask')
      mask Help: eval('openHelp(209)')
      mask Display: image(imread('HeadLight.png'))
  TrafficLightRoadSideNL_2_Red : Subsystem  Tag=actuator/Red  Priority=0  LoadFcn=load('PreScanVisuLightActuatorData');load('PrescanRPYData');load('PrescanXYZData');load('PreScanRGBData')  mask(PreScan Sink Block: VisuActiveLight){}
      mask help:
      | The VisuActiveLight block provides a way for detailed animation of Light Sources, such as the indicator, brake, fog and main lights of a vehicle, or a light post.
      |
      | For more information, please click Help.
      settings: OpenFcn=open_system([gcb '/Actuator'],'mask')
      mask Help: eval('openHelp(209)')
      mask Display: image(imread('HeadLight.png'))
  TrafficLightRoadSideNL_3 : Subsystem  Tag=WorldObjectSubSystem  InitFcn=UniqueId = '649';
      mask init: same as W01_Base_MapUnrealPb_cs/TrafficLightRoadSideNL_1
      mask Display: image(imread(imagePath));color('white');text(0, 0, ' ID=78\n')
  TrafficLightRoadSideNL_3_Green : Subsystem  Tag=actuator/Green  Priority=0  LoadFcn=load('PreScanVisuLightActuatorData');load('PrescanRPYData');load('PrescanXYZData');load('PreScanRGBData')  mask(PreScan Sink Block: VisuActiveLight){}
      mask help:
      | The VisuActiveLight block provides a way for detailed animation of Light Sources, such as the indicator, brake, fog and main lights of a vehicle, or a light post.
      |
      | For more information, please click Help.
      settings: OpenFcn=open_system([gcb '/Actuator'],'mask')
      mask Help: eval('openHelp(209)')
      mask Display: image(imread('HeadLight.png'))
  TrafficLightRoadSideNL_3_Orange : Subsystem  Tag=actuator/Orange  Priority=0  LoadFcn=load('PreScanVisuLightActuatorData');load('PrescanRPYData');load('PrescanXYZData');load('PreScanRGBData')  mask(PreScan Sink Block: VisuActiveLight){}
      mask help:
      | The VisuActiveLight block provides a way for detailed animation of Light Sources, such as the indicator, brake, fog and main lights of a vehicle, or a light post.
      |
      | For more information, please click Help.
      settings: OpenFcn=open_system([gcb '/Actuator'],'mask')
      mask Help: eval('openHelp(209)')
      mask Display: image(imread('HeadLight.png'))
  TrafficLightRoadSideNL_3_Red : Subsystem  Tag=actuator/Red  Priority=0  LoadFcn=load('PreScanVisuLightActuatorData');load('PrescanRPYData');load('PrescanXYZData');load('PreScanRGBData')  mask(PreScan Sink Block: VisuActiveLight){}
      mask help:
      | The VisuActiveLight block provides a way for detailed animation of Light Sources, such as the indicator, brake, fog and main lights of a vehicle, or a light post.
      |
      | For more information, please click Help.
      settings: OpenFcn=open_system([gcb '/Actuator'],'mask')
      mask Help: eval('openHelp(209)')
      mask Display: image(imread('HeadLight.png'))
  TrafficLightRoadSideNL_4 : Subsystem  Tag=WorldObjectSubSystem  InitFcn=UniqueId = '650';
      mask init: same as W01_Base_MapUnrealPb_cs/TrafficLightRoadSideNL_1
      mask Display: image(imread(imagePath));color('white');text(0, 0, ' ID=79\n')
  TrafficLightRoadSideNL_4_Green : Subsystem  Tag=actuator/Green  Priority=0  LoadFcn=load('PreScanVisuLightActuatorData');load('PrescanRPYData');load('PrescanXYZData');load('PreScanRGBData')  mask(PreScan Sink Block: VisuActiveLight){}
      mask help:
      | The VisuActiveLight block provides a way for detailed animation of Light Sources, such as the indicator, brake, fog and main lights of a vehicle, or a light post.
      |
      | For more information, please click Help.
      settings: OpenFcn=open_system([gcb '/Actuator'],'mask')
      mask Help: eval('openHelp(209)')
      mask Display: image(imread('HeadLight.png'))
  TrafficLightRoadSideNL_4_Orange : Subsystem  Tag=actuator/Orange  Priority=0  LoadFcn=load('PreScanVisuLightActuatorData');load('PrescanRPYData');load('PrescanXYZData');load('PreScanRGBData')  mask(PreScan Sink Block: VisuActiveLight){}
      mask help:
      | The VisuActiveLight block provides a way for detailed animation of Light Sources, such as the indicator, brake, fog and main lights of a vehicle, or a light post.
      |
      | For more information, please click Help.
      settings: OpenFcn=open_system([gcb '/Actuator'],'mask')
      mask Help: eval('openHelp(209)')
      mask Display: image(imread('HeadLight.png'))
  TrafficLightRoadSideNL_4_Red : Subsystem  Tag=actuator/Red  Priority=0  LoadFcn=load('PreScanVisuLightActuatorData');load('PrescanRPYData');load('PrescanXYZData');load('PreScanRGBData')  mask(PreScan Sink Block: VisuActiveLight){}
      mask help:
      | The VisuActiveLight block provides a way for detailed animation of Light Sources, such as the indicator, brake, fog and main lights of a vehicle, or a light post.
      |
      | For more information, please click Help.
      settings: OpenFcn=open_system([gcb '/Actuator'],'mask')
      mask Help: eval('openHelp(209)')
      mask Display: image(imread('HeadLight.png'))
  TrafficLightRoadSideNL_5 : Subsystem  Tag=WorldObjectSubSystem  InitFcn=UniqueId = '651';
      mask init: same as W01_Base_MapUnrealPb_cs/TrafficLightRoadSideNL_1
      mask Display: image(imread(imagePath));color('white');text(0, 0, ' ID=80\n')
  TrafficLightRoadSideNL_5_Green : Subsystem  Tag=actuator/Green  Priority=0  LoadFcn=load('PreScanVisuLightActuatorData');load('PrescanRPYData');load('PrescanXYZData');load('PreScanRGBData')  mask(PreScan Sink Block: VisuActiveLight){}
      mask help:
      | The VisuActiveLight block provides a way for detailed animation of Light Sources, such as the indicator, brake, fog and main lights of a vehicle, or a light post.
      |
      | For more information, please click Help.
      settings: OpenFcn=open_system([gcb '/Actuator'],'mask')
      mask Help: eval('openHelp(209)')
      mask Display: image(imread('HeadLight.png'))
  TrafficLightRoadSideNL_5_Orange : Subsystem  Tag=actuator/Orange  Priority=0  LoadFcn=load('PreScanVisuLightActuatorData');load('PrescanRPYData');load('PrescanXYZData');load('PreScanRGBData')  mask(PreScan Sink Block: VisuActiveLight){}
      mask help:
      | The VisuActiveLight block provides a way for detailed animation of Light Sources, such as the indicator, brake, fog and main lights of a vehicle, or a light post.
      |
      | For more information, please click Help.
      settings: OpenFcn=open_system([gcb '/Actuator'],'mask')
      mask Help: eval('openHelp(209)')
      mask Display: image(imread('HeadLight.png'))
  TrafficLightRoadSideNL_5_Red : Subsystem  Tag=actuator/Red  Priority=0  LoadFcn=load('PreScanVisuLightActuatorData');load('PrescanRPYData');load('PrescanXYZData');load('PreScanRGBData')  mask(PreScan Sink Block: VisuActiveLight){}
      mask help:
      | The VisuActiveLight block provides a way for detailed animation of Light Sources, such as the indicator, brake, fog and main lights of a vehicle, or a light post.
      |
      | For more information, please click Help.
      settings: OpenFcn=open_system([gcb '/Actuator'],'mask')
      mask Help: eval('openHelp(209)')
      mask Display: image(imread('HeadLight.png'))
  TrafficLightRoadSideNL_6 : Subsystem  Tag=WorldObjectSubSystem  InitFcn=UniqueId = '10446';
      mask init: same as W01_Base_MapUnrealPb_cs/TrafficLightRoadSideNL_1
      mask Display: image(imread(imagePath));color('white');text(0, 0, ' ID=81\n')
  TrafficLightRoadSideNL_6_Green : Subsystem  Tag=actuator/Green  Priority=0  LoadFcn=load('PreScanVisuLightActuatorData');load('PrescanRPYData');load('PrescanXYZData');load('PreScanRGBData')  mask(PreScan Sink Block: VisuActiveLight){}
      mask help:
      | The VisuActiveLight block provides a way for detailed animation of Light Sources, such as the indicator, brake, fog and main lights of a vehicle, or a light post.
      |
      | For more information, please click Help.
      settings: OpenFcn=open_system([gcb '/Actuator'],'mask')
      mask Help: eval('openHelp(209)')
      mask Display: image(imread('HeadLight.png'))
  TrafficLightRoadSideNL_6_Orange : Subsystem  Tag=actuator/Orange  Priority=0  LoadFcn=load('PreScanVisuLightActuatorData');load('PrescanRPYData');load('PrescanXYZData');load('PreScanRGBData')  mask(PreScan Sink Block: VisuActiveLight){}
      mask help:
      | The VisuActiveLight block provides a way for detailed animation of Light Sources, such as the indicator, brake, fog and main lights of a vehicle, or a light post.
      |
      | For more information, please click Help.
      settings: OpenFcn=open_system([gcb '/Actuator'],'mask')
      mask Help: eval('openHelp(209)')
      mask Display: image(imread('HeadLight.png'))
  TrafficLightRoadSideNL_6_Red : Subsystem  Tag=actuator/Red  Priority=0  LoadFcn=load('PreScanVisuLightActuatorData');load('PrescanRPYData');load('PrescanXYZData');load('PreScanRGBData')  mask(PreScan Sink Block: VisuActiveLight){}
      mask help:
      | The VisuActiveLight block provides a way for detailed animation of Light Sources, such as the indicator, brake, fog and main lights of a vehicle, or a light post.
      |
      | For more information, please click Help.
      settings: OpenFcn=open_system([gcb '/Actuator'],'mask')
      mask Help: eval('openHelp(209)')
      mask Display: image(imread('HeadLight.png'))
  TrafficLightRoadSideNL_7 : Subsystem  Tag=WorldObjectSubSystem  InitFcn=UniqueId = '653';
      mask init: same as W01_Base_MapUnrealPb_cs/TrafficLightRoadSideNL_1
      mask Display: image(imread(imagePath));color('white');text(0, 0, ' ID=82\n')
  TrafficLightRoadSideNL_7_Green : Subsystem  Tag=actuator/Green  Priority=0  LoadFcn=load('PreScanVisuLightActuatorData');load('PrescanRPYData');load('PrescanXYZData');load('PreScanRGBData')  mask(PreScan Sink Block: VisuActiveLight){}
      mask help:
      | The VisuActiveLight block provides a way for detailed animation of Light Sources, such as the indicator, brake, fog and main lights of a vehicle, or a light post.
      |
      | For more information, please click Help.
      settings: OpenFcn=open_system([gcb '/Actuator'],'mask')
      mask Help: eval('openHelp(209)')
      mask Display: image(imread('HeadLight.png'))
  TrafficLightRoadSideNL_7_Orange : Subsystem  Tag=actuator/Orange  Priority=0  LoadFcn=load('PreScanVisuLightActuatorData');load('PrescanRPYData');load('PrescanXYZData');load('PreScanRGBData')  mask(PreScan Sink Block: VisuActiveLight){}
      mask help:
      | The VisuActiveLight block provides a way for detailed animation of Light Sources, such as the indicator, brake, fog and main lights of a vehicle, or a light post.
      |
      | For more information, please click Help.
      settings: OpenFcn=open_system([gcb '/Actuator'],'mask')
      mask Help: eval('openHelp(209)')
      mask Display: image(imread('HeadLight.png'))
  TrafficLightRoadSideNL_7_Red : Subsystem  Tag=actuator/Red  Priority=0  LoadFcn=load('PreScanVisuLightActuatorData');load('PrescanRPYData');load('PrescanXYZData');load('PreScanRGBData')  mask(PreScan Sink Block: VisuActiveLight){}
      mask help:
      | The VisuActiveLight block provides a way for detailed animation of Light Sources, such as the indicator, brake, fog and main lights of a vehicle, or a light post.
      |
      | For more information, please click Help.
      settings: OpenFcn=open_system([gcb '/Actuator'],'mask')
      mask Help: eval('openHelp(209)')
      mask Display: image(imread('HeadLight.png'))
  TrafficLightRoadSideNL_8 : Subsystem  Tag=WorldObjectSubSystem  InitFcn=UniqueId = '654';
      mask init: same as W01_Base_MapUnrealPb_cs/TrafficLightRoadSideNL_1
      mask Display: image(imread(imagePath));color('white');text(0, 0, ' ID=83\n')
  TrafficLightRoadSideNL_8_Green : Subsystem  Tag=actuator/Green  Priority=0  LoadFcn=load('PreScanVisuLightActuatorData');load('PrescanRPYData');load('PrescanXYZData');load('PreScanRGBData')  mask(PreScan Sink Block: VisuActiveLight){}
      mask help:
      | The VisuActiveLight block provides a way for detailed animation of Light Sources, such as the indicator, brake, fog and main lights of a vehicle, or a light post.
      |
      | For more information, please click Help.
      settings: OpenFcn=open_system([gcb '/Actuator'],'mask')
      mask Help: eval('openHelp(209)')
      mask Display: image(imread('HeadLight.png'))
  TrafficLightRoadSideNL_8_Orange : Subsystem  Tag=actuator/Orange  Priority=0  LoadFcn=load('PreScanVisuLightActuatorData');load('PrescanRPYData');load('PrescanXYZData');load('PreScanRGBData')  mask(PreScan Sink Block: VisuActiveLight){}
      mask help:
      | The VisuActiveLight block provides a way for detailed animation of Light Sources, such as the indicator, brake, fog and main lights of a vehicle, or a light post.
      |
      | For more information, please click Help.
      settings: OpenFcn=open_system([gcb '/Actuator'],'mask')
      mask Help: eval('openHelp(209)')
      mask Display: image(imread('HeadLight.png'))
  TrafficLightRoadSideNL_8_Red : Subsystem  Tag=actuator/Red  Priority=0  LoadFcn=load('PreScanVisuLightActuatorData');load('PrescanRPYData');load('PrescanXYZData');load('PreScanRGBData')  mask(PreScan Sink Block: VisuActiveLight){}
      mask help:
      | The VisuActiveLight block provides a way for detailed animation of Light Sources, such as the indicator, brake, fog and main lights of a vehicle, or a light post.
      |
      | For more information, please click Help.
      settings: OpenFcn=open_system([gcb '/Actuator'],'mask')
      mask Help: eval('openHelp(209)')
      mask Display: image(imread('HeadLight.png'))
  VISUColorRegion_Lower_Body_Child_RegularAni_1 : Subsystem  Tag=actuator/ColorRegion  Priority=0  LoadFcn=load('PrescanColorData')  mask(PreScan Sink Block: VisuTextureColor){}
      mask help:
      | The VisuTextureColor block provides a way to adapt the color of a vehicle.
      |
      | For more information, please click Help.
      settings: OpenFcn=open_system([gcb '/Actuator'],'mask')
      mask Help: eval('openHelp(230)')
      mask Display: image(imread('TextureColor.png'))
  VISUColorRegion_Lower_Body_Child_RegularAni_2 : Subsystem  Tag=actuator/ColorRegion  Priority=0  LoadFcn=load('PrescanColorData')  mask(PreScan Sink Block: VisuTextureColor){}
      mask help:
      | The VisuTextureColor block provides a way to adapt the color of a vehicle.
      |
      | For more information, please click Help.
      settings: OpenFcn=open_system([gcb '/Actuator'],'mask')
      mask Help: eval('openHelp(230)')
      mask Display: image(imread('TextureColor.png'))
  VISUColorRegion_Lower_Body_Female_RegularAni_1 : Subsystem  Tag=actuator/ColorRegion  Priority=0  LoadFcn=load('PrescanColorData')  mask(PreScan Sink Block: VisuTextureColor){}
      mask help:
      | The VisuTextureColor block provides a way to adapt the color of a vehicle.
      |
      | For more information, please click Help.
      settings: OpenFcn=open_system([gcb '/Actuator'],'mask')
      mask Help: eval('openHelp(230)')
      mask Display: image(imread('TextureColor.png'))
  VISUColorRegion_Lower_Body_Male_RegularAni_1 : Subsystem  Tag=actuator/ColorRegion  Priority=0  LoadFcn=load('PrescanColorData')  mask(PreScan Sink Block: VisuTextureColor){}
      mask help:
      | The VisuTextureColor block provides a way to adapt the color of a vehicle.
      |
      | For more information, please click Help.
      settings: OpenFcn=open_system([gcb '/Actuator'],'mask')
      mask Help: eval('openHelp(230)')
      mask Display: image(imread('TextureColor.png'))
  VISUColorRegion_Lower_Body_Male_RegularAni_2 : Subsystem  Tag=actuator/ColorRegion  Priority=0  LoadFcn=load('PrescanColorData')  mask(PreScan Sink Block: VisuTextureColor){}
      mask help:
      | The VisuTextureColor block provides a way to adapt the color of a vehicle.
      |
      | For more information, please click Help.
      settings: OpenFcn=open_system([gcb '/Actuator'],'mask')
      mask Help: eval('openHelp(230)')
      mask Display: image(imread('TextureColor.png'))
  VISUColorRegion_Shoes_Child_RegularAni_1 : Subsystem  Tag=actuator/ColorRegion  Priority=0  LoadFcn=load('PrescanColorData')  mask(PreScan Sink Block: VisuTextureColor){}
      mask help:
      | The VisuTextureColor block provides a way to adapt the color of a vehicle.
      |
      | For more information, please click Help.
      settings: OpenFcn=open_system([gcb '/Actuator'],'mask')
      mask Help: eval('openHelp(230)')
      mask Display: image(imread('TextureColor.png'))
  VISUColorRegion_Shoes_Child_RegularAni_2 : Subsystem  Tag=actuator/ColorRegion  Priority=0  LoadFcn=load('PrescanColorData')  mask(PreScan Sink Block: VisuTextureColor){}
      mask help:
      | The VisuTextureColor block provides a way to adapt the color of a vehicle.
      |
      | For more information, please click Help.
      settings: OpenFcn=open_system([gcb '/Actuator'],'mask')
      mask Help: eval('openHelp(230)')
      mask Display: image(imread('TextureColor.png'))
  VISUColorRegion_Shoes_Female_RegularAni_1 : Subsystem  Tag=actuator/ColorRegion  Priority=0  LoadFcn=load('PrescanColorData')  mask(PreScan Sink Block: VisuTextureColor){}
      mask help:
      | The VisuTextureColor block provides a way to adapt the color of a vehicle.
      |
      | For more information, please click Help.
      settings: OpenFcn=open_system([gcb '/Actuator'],'mask')
      mask Help: eval('openHelp(230)')
      mask Display: image(imread('TextureColor.png'))
  VISUColorRegion_Shoes_Male_RegularAni_1 : Subsystem  Tag=actuator/ColorRegion  Priority=0  LoadFcn=load('PrescanColorData')  mask(PreScan Sink Block: VisuTextureColor){}
      mask help:
      | The VisuTextureColor block provides a way to adapt the color of a vehicle.
      |
      | For more information, please click Help.
      settings: OpenFcn=open_system([gcb '/Actuator'],'mask')
      mask Help: eval('openHelp(230)')
      mask Display: image(imread('TextureColor.png'))
  VISUColorRegion_Shoes_Male_RegularAni_2 : Subsystem  Tag=actuator/ColorRegion  Priority=0  LoadFcn=load('PrescanColorData')  mask(PreScan Sink Block: VisuTextureColor){}
      mask help:
      | The VisuTextureColor block provides a way to adapt the color of a vehicle.
      |
      | For more information, please click Help.
      settings: OpenFcn=open_system([gcb '/Actuator'],'mask')
      mask Help: eval('openHelp(230)')
      mask Display: image(imread('TextureColor.png'))
  VISUColorRegion_Upper_Body_Child_RegularAni_1 : Subsystem  Tag=actuator/ColorRegion  Priority=0  LoadFcn=load('PrescanColorData')  mask(PreScan Sink Block: VisuTextureColor){}
      mask help:
      | The VisuTextureColor block provides a way to adapt the color of a vehicle.
      |
      | For more information, please click Help.
      settings: OpenFcn=open_system([gcb '/Actuator'],'mask')
      mask Help: eval('openHelp(230)')
      mask Display: image(imread('TextureColor.png'))
  VISUColorRegion_Upper_Body_Child_RegularAni_2 : Subsystem  Tag=actuator/ColorRegion  Priority=0  LoadFcn=load('PrescanColorData')  mask(PreScan Sink Block: VisuTextureColor){}
      mask help:
      | The VisuTextureColor block provides a way to adapt the color of a vehicle.
      |
      | For more information, please click Help.
      settings: OpenFcn=open_system([gcb '/Actuator'],'mask')
      mask Help: eval('openHelp(230)')
      mask Display: image(imread('TextureColor.png'))
  VISUColorRegion_Upper_Body_Female_RegularAni_1 : Subsystem  Tag=actuator/ColorRegion  Priority=0  LoadFcn=load('PrescanColorData')  mask(PreScan Sink Block: VisuTextureColor){}
      mask help:
      | The VisuTextureColor block provides a way to adapt the color of a vehicle.
      |
      | For more information, please click Help.
      settings: OpenFcn=open_system([gcb '/Actuator'],'mask')
      mask Help: eval('openHelp(230)')
      mask Display: image(imread('TextureColor.png'))
  VISUColorRegion_Upper_Body_Male_RegularAni_1 : Subsystem  Tag=actuator/ColorRegion  Priority=0  LoadFcn=load('PrescanColorData')  mask(PreScan Sink Block: VisuTextureColor){}
      mask help:
      | The VisuTextureColor block provides a way to adapt the color of a vehicle.
      |
      | For more information, please click Help.
      settings: OpenFcn=open_system([gcb '/Actuator'],'mask')
      mask Help: eval('openHelp(230)')
      mask Display: image(imread('TextureColor.png'))
  VISUColorRegion_Upper_Body_Male_RegularAni_2 : Subsystem  Tag=actuator/ColorRegion  Priority=0  LoadFcn=load('PrescanColorData')  mask(PreScan Sink Block: VisuTextureColor){}
      mask help:
      | The VisuTextureColor block provides a way to adapt the color of a vehicle.
      |
      | For more information, please click Help.
      settings: OpenFcn=open_system([gcb '/Actuator'],'mask')
      mask Help: eval('openHelp(230)')
      mask Display: image(imread('TextureColor.png'))
  Vector Concatenate : Concatenate  NumInputs=3
  pose_otheCar : Subsystem
  wires:
  [other] -> pose_otheCar/Enable
  Vector Concatenate/1 -> pose_otheCar/1(In1)
  Audi_A8_Sedan_1/2(SafetyPlannerLoc) -> Vector Concatenate/2
  Citroen_C3_Hatchback_1/2(SafetyPlannerLoc) -> Vector Concatenate/3
  BMW_X5_SUV_1/1(STATE_BMW_X5_SUV_1_bus) -> STATE_BMW_X5_SUV_1_bus/1(STATE_BMW_X5_SUV_1_bus)
  SELF_BMW_X5_SUV_1/1(SELF_BMW_X5_SUV_1) -> BMW_X5_SUV_1/1(SELF_BMW_X5_SUV_1)
  Radar_1/1(Radar_1) -> BMW_X5_SUV_1/2(Radar_1)
  PointCloudSensor_1/1(PointCloudSensor_1) -> BMW_X5_SUV_1/3(PointCloudSensor_1)
  PointCloudSensor_2/1(PointCloudSensor_2) -> BMW_X5_SUV_1/4(PointCloudSensor_2)
  PointCloudSensor_3/1(PointCloudSensor_3) -> BMW_X5_SUV_1/5(PointCloudSensor_3)
  PointCloudSensor_4/1(PointCloudSensor_4) -> BMW_X5_SUV_1/6(PointCloudSensor_4)
  PhysicsBasedCameraUnreal_1_ImageRGBOutput_image/1(PhysicsBasedCameraUnreal_1_ImageRGBOutput_image) -> BMW_X5_SUV_1/7(PhysicsBasedCameraUnreal_1_ImageRGBOutput_image)
  PhysicsBasedCameraUnreal_2_ImageRGBOutput_image/1(PhysicsBasedCameraUnreal_2_ImageRGBOutput_image) -> BMW_X5_SUV_1/8(PhysicsBasedCameraUnreal_2_ImageRGBOutput_image)
  PhysicsBasedCameraUnreal_3_ImageRGBOutput_image/1(PhysicsBasedCameraUnreal_3_ImageRGBOutput_image) -> BMW_X5_SUV_1/9(PhysicsBasedCameraUnreal_3_ImageRGBOutput_image)
  BMW_X5_SUV_1/2(PhysicsBasedCameraUnreal_1_PBCUPose_Control) -> PhysicsBasedCameraUnreal_1_PBCUPose_Control/1(PhysicsBasedCameraUnreal_1_PBCUPose_Control)
  BMW_X5_SUV_1/3(PhysicsBasedCameraUnreal_1_PBCUExposure_Control) -> PhysicsBasedCameraUnreal_1_PBCUExposure_Control/1(PhysicsBasedCameraUnreal_1_PBCUExposure_Control)
  BMW_X5_SUV_1/4(PhysicsBasedCameraUnreal_2_PBCUPose_Control) -> PhysicsBasedCameraUnreal_2_PBCUPose_Control/1(PhysicsBasedCameraUnreal_2_PBCUPose_Control)
  BMW_X5_SUV_1/5(PhysicsBasedCameraUnreal_2_PBCUExposure_Control) -> PhysicsBasedCameraUnreal_2_PBCUExposure_Control/1(PhysicsBasedCameraUnreal_2_PBCUExposure_Control)
  BMW_X5_SUV_1/6(PhysicsBasedCameraUnreal_3_PBCUPose_Control) -> PhysicsBasedCameraUnreal_3_PBCUPose_Control/1(PhysicsBasedCameraUnreal_3_PBCUPose_Control)
  BMW_X5_SUV_1/7(PhysicsBasedCameraUnreal_3_PBCUExposure_Control) -> PhysicsBasedCameraUnreal_3_PBCUExposure_Control/1(PhysicsBasedCameraUnreal_3_PBCUExposure_Control)
  Audi_A8_Sedan_1/1(STATE_Audi_A8_Sedan_1_bus) -> STATE_Audi_A8_Sedan_1_bus/1(STATE_Audi_A8_Sedan_1_bus)
  SELF_Audi_A8_Sedan_1/1(SELF_Audi_A8_Sedan_1) -> Audi_A8_Sedan_1/1(SELF_Audi_A8_Sedan_1)
  Citroen_C3_Hatchback_1/1(STATE_Citroen_C3_Hatchback_1_bus) -> STATE_Citroen_C3_Hatchback_1_bus/1(STATE_Citroen_C3_Hatchback_1_bus)
  SELF_Citroen_C3_Hatchback_1/1(SELF_Citroen_C3_Hatchback_1) -> Citroen_C3_Hatchback_1/1(SELF_Citroen_C3_Hatchback_1)
  TrafficLightRoadSideNL_1/1(TrafficLightRoadSideNL_1_Red) -> TrafficLightRoadSideNL_1_Red/1(TrafficLightRoadSideNL_1_Red)
  TrafficLightRoadSideNL_1/2(TrafficLightRoadSideNL_1_Orange) -> TrafficLightRoadSideNL_1_Orange/1(TrafficLightRoadSideNL_1_Orange)
  TrafficLightRoadSideNL_1/3(TrafficLightRoadSideNL_1_Green) -> TrafficLightRoadSideNL_1_Green/1(TrafficLightRoadSideNL_1_Green)
  TrafficLightRoadSideNL_2/1(TrafficLightRoadSideNL_2_Red) -> TrafficLightRoadSideNL_2_Red/1(TrafficLightRoadSideNL_2_Red)
  TrafficLightRoadSideNL_2/2(TrafficLightRoadSideNL_2_Orange) -> TrafficLightRoadSideNL_2_Orange/1(TrafficLightRoadSideNL_2_Orange)
  TrafficLightRoadSideNL_2/3(TrafficLightRoadSideNL_2_Green) -> TrafficLightRoadSideNL_2_Green/1(TrafficLightRoadSideNL_2_Green)
  TrafficLightRoadSideNL_3/1(TrafficLightRoadSideNL_3_Red) -> TrafficLightRoadSideNL_3_Red/1(TrafficLightRoadSideNL_3_Red)
  TrafficLightRoadSideNL_3/2(TrafficLightRoadSideNL_3_Orange) -> TrafficLightRoadSideNL_3_Orange/1(TrafficLightRoadSideNL_3_Orange)
  TrafficLightRoadSideNL_3/3(TrafficLightRoadSideNL_3_Green) -> TrafficLightRoadSideNL_3_Green/1(TrafficLightRoadSideNL_3_Green)
  TrafficLightRoadSideNL_4/1(TrafficLightRoadSideNL_4_Red) -> TrafficLightRoadSideNL_4_Red/1(TrafficLightRoadSideNL_4_Red)
  TrafficLightRoadSideNL_4/2(TrafficLightRoadSideNL_4_Orange) -> TrafficLightRoadSideNL_4_Orange/1(TrafficLightRoadSideNL_4_Orange)
  TrafficLightRoadSideNL_4/3(TrafficLightRoadSideNL_4_Green) -> TrafficLightRoadSideNL_4_Green/1(TrafficLightRoadSideNL_4_Green)
  TrafficLightRoadSideNL_5/1(TrafficLightRoadSideNL_5_Red) -> TrafficLightRoadSideNL_5_Red/1(TrafficLightRoadSideNL_5_Red)
  TrafficLightRoadSideNL_5/2(TrafficLightRoadSideNL_5_Orange) -> TrafficLightRoadSideNL_5_Orange/1(TrafficLightRoadSideNL_5_Orange)
  TrafficLightRoadSideNL_5/3(TrafficLightRoadSideNL_5_Green) -> TrafficLightRoadSideNL_5_Green/1(TrafficLightRoadSideNL_5_Green)
  TrafficLightRoadSideNL_7/1(TrafficLightRoadSideNL_7_Red) -> TrafficLightRoadSideNL_7_Red/1(TrafficLightRoadSideNL_7_Red)
  TrafficLightRoadSideNL_7/2(TrafficLightRoadSideNL_7_Orange) -> TrafficLightRoadSideNL_7_Orange/1(TrafficLightRoadSideNL_7_Orange)
  TrafficLightRoadSideNL_7/3(TrafficLightRoadSideNL_7_Green) -> TrafficLightRoadSideNL_7_Green/1(TrafficLightRoadSideNL_7_Green)
  TrafficLightRoadSideNL_8/1(TrafficLightRoadSideNL_8_Red) -> TrafficLightRoadSideNL_8_Red/1(TrafficLightRoadSideNL_8_Red)
  TrafficLightRoadSideNL_8/2(TrafficLightRoadSideNL_8_Orange) -> TrafficLightRoadSideNL_8_Orange/1(TrafficLightRoadSideNL_8_Orange)
  TrafficLightRoadSideNL_8/3(TrafficLightRoadSideNL_8_Green) -> TrafficLightRoadSideNL_8_Green/1(TrafficLightRoadSideNL_8_Green)
  TrafficLightRoadSideNL_6/1(TrafficLightRoadSideNL_6_Red) -> TrafficLightRoadSideNL_6_Red/1(TrafficLightRoadSideNL_6_Red)
  TrafficLightRoadSideNL_6/2(TrafficLightRoadSideNL_6_Orange) -> TrafficLightRoadSideNL_6_Orange/1(TrafficLightRoadSideNL_6_Orange)
  TrafficLightRoadSideNL_6/3(TrafficLightRoadSideNL_6_Green) -> TrafficLightRoadSideNL_6_Green/1(TrafficLightRoadSideNL_6_Green)
  Child_RegularAni_1/1(STATE_Child_RegularAni_1_bus) -> STATE_Child_RegularAni_1_bus/1(STATE_Child_RegularAni_1_bus)
  Child_RegularAni_1/2(ANIM_Child_RegularAni_1) -> ANIM_Child_RegularAni_1/1(ANIM_Child_RegularAni_1)
  SELF_Child_RegularAni_1/1(SELF_Child_RegularAni_1) -> Child_RegularAni_1/1(SELF_Child_RegularAni_1)
  Child_RegularAni_1/3(VISUColorRegion_Upper_Body_Child_RegularAni_1) -> VISUColorRegion_Upper_Body_Child_RegularAni_1/1(VISUColorRegion_Upper_Body_Child_RegularAni_1)
  Child_RegularAni_1/4(VISUColorRegion_Lower_Body_Child_RegularAni_1) -> VISUColorRegion_Lower_Body_Child_RegularAni_1/1(VISUColorRegion_Lower_Body_Child_RegularAni_1)
  Child_RegularAni_1/5(VISUColorRegion_Shoes_Child_RegularAni_1) -> VISUColorRegion_Shoes_Child_RegularAni_1/1(VISUColorRegion_Shoes_Child_RegularAni_1)
  Child_RegularAni_2/1(STATE_Child_RegularAni_2_bus) -> STATE_Child_RegularAni_2_bus/1(STATE_Child_RegularAni_2_bus)
  Child_RegularAni_2/2(ANIM_Child_RegularAni_2) -> ANIM_Child_RegularAni_2/1(ANIM_Child_RegularAni_2)
  SELF_Child_RegularAni_2/1(SELF_Child_RegularAni_2) -> Child_RegularAni_2/1(SELF_Child_RegularAni_2)
  Child_RegularAni_2/3(VISUColorRegion_Upper_Body_Child_RegularAni_2) -> VISUColorRegion_Upper_Body_Child_RegularAni_2/1(VISUColorRegion_Upper_Body_Child_RegularAni_2)
  Child_RegularAni_2/4(VISUColorRegion_Lower_Body_Child_RegularAni_2) -> VISUColorRegion_Lower_Body_Child_RegularAni_2/1(VISUColorRegion_Lower_Body_Child_RegularAni_2)
  Child_RegularAni_2/5(VISUColorRegion_Shoes_Child_RegularAni_2) -> VISUColorRegion_Shoes_Child_RegularAni_2/1(VISUColorRegion_Shoes_Child_RegularAni_2)
  Female_RegularAni_1/1(STATE_Female_RegularAni_1_bus) -> STATE_Female_RegularAni_1_bus/1(STATE_Female_RegularAni_1_bus)
  Female_RegularAni_1/2(ANIM_Female_RegularAni_1) -> ANIM_Female_RegularAni_1/1(ANIM_Female_RegularAni_1)
  SELF_Female_RegularAni_1/1(SELF_Female_RegularAni_1) -> Female_RegularAni_1/1(SELF_Female_RegularAni_1)
  Female_RegularAni_1/3(VISUColorRegion_Upper_Body_Female_RegularAni_1) -> VISUColorRegion_Upper_Body_Female_RegularAni_1/1(VISUColorRegion_Upper_Body_Female_RegularAni_1)
  Female_RegularAni_1/4(VISUColorRegion_Lower_Body_Female_RegularAni_1) -> VISUColorRegion_Lower_Body_Female_RegularAni_1/1(VISUColorRegion_Lower_Body_Female_RegularAni_1)
  Female_RegularAni_1/5(VISUColorRegion_Shoes_Female_RegularAni_1) -> VISUColorRegion_Shoes_Female_RegularAni_1/1(VISUColorRegion_Shoes_Female_RegularAni_1)
  Male_RegularAni_1/1(STATE_Male_RegularAni_1_bus) -> STATE_Male_RegularAni_1_bus/1(STATE_Male_RegularAni_1_bus)
  Male_RegularAni_1/2(ANIM_Male_RegularAni_1) -> ANIM_Male_RegularAni_1/1(ANIM_Male_RegularAni_1)
  SELF_Male_RegularAni_1/1(SELF_Male_RegularAni_1) -> Male_RegularAni_1/1(SELF_Male_RegularAni_1)
  Male_RegularAni_1/3(VISUColorRegion_Upper_Body_Male_RegularAni_1) -> VISUColorRegion_Upper_Body_Male_RegularAni_1/1(VISUColorRegion_Upper_Body_Male_RegularAni_1)
  Male_RegularAni_1/4(VISUColorRegion_Lower_Body_Male_RegularAni_1) -> VISUColorRegion_Lower_Body_Male_RegularAni_1/1(VISUColorRegion_Lower_Body_Male_RegularAni_1)
  Male_RegularAni_1/5(VISUColorRegion_Shoes_Male_RegularAni_1) -> VISUColorRegion_Shoes_Male_RegularAni_1/1(VISUColorRegion_Shoes_Male_RegularAni_1)
  Male_RegularAni_2/1(STATE_Male_RegularAni_2_bus) -> STATE_Male_RegularAni_2_bus/1(STATE_Male_RegularAni_2_bus)
  Male_RegularAni_2/2(ANIM_Male_RegularAni_2) -> ANIM_Male_RegularAni_2/1(ANIM_Male_RegularAni_2)
  SELF_Male_RegularAni_2/1(SELF_Male_RegularAni_2) -> Male_RegularAni_2/1(SELF_Male_RegularAni_2)
  Male_RegularAni_2/3(VISUColorRegion_Upper_Body_Male_RegularAni_2) -> VISUColorRegion_Upper_Body_Male_RegularAni_2/1(VISUColorRegion_Upper_Body_Male_RegularAni_2)
  Male_RegularAni_2/4(VISUColorRegion_Lower_Body_Male_RegularAni_2) -> VISUColorRegion_Lower_Body_Male_RegularAni_2/1(VISUColorRegion_Lower_Body_Male_RegularAni_2)
  Male_RegularAni_2/5(VISUColorRegion_Shoes_Male_RegularAni_2) -> VISUColorRegion_Shoes_Male_RegularAni_2/1(VISUColorRegion_Shoes_Male_RegularAni_2)
  Ground_1/1 -> Vector Concatenate/1
